simulink model "Rider_Controls_Full_CAN_Enable"  (R2014b)
settings: configuration reference "Embedded_Configuration" (kept outside this file)
PreLoadFcn:
  | load('Embedded_Config.mat')
PostLoadFcn:
  | c2000demoscallback(1)
model workspace: external: MAT-File Embedded_Config.mat (data not in the file)
libraries: canmsglib x2, c280xlib x2
settings Model: Creator=The MathWorks Inc.  LastModifiedBy=Sean

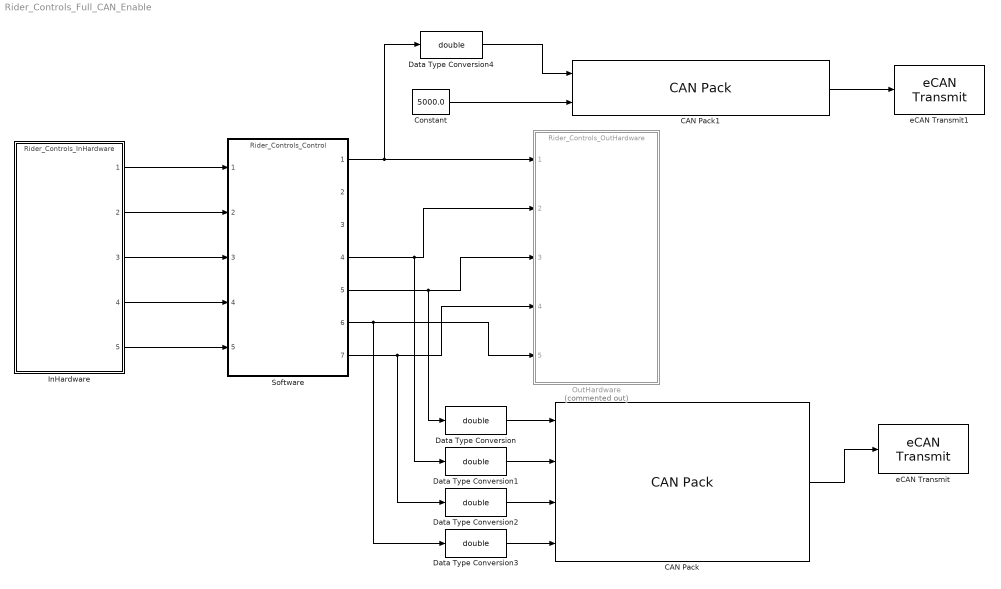
== system Rider_Controls_Full_CAN_Enable ==
  CAN Pack : canmsglib/CAN Pack  CANdbFile=C:\Users\Sean\Desktop\Buckeye Current\Databases\RW3.dbc  MsgList=DriveControlsLimits  MsgName=DriveControlsLimits  MsgIDType=Standard (11-bit identifier)  MsgIdentifier=483  MsgLength=8  SignalInfo=BatteryLimit$1$1$1$2$1$0$1$0$0$1$#RPMLimit$2$1$1$2$1$0$1$0$0$1$#StatusLimit$3$1$1$2$1$0$1$0$-Inf$Inf$#ThrottleLock$0$1$1$2$1$0$1$0$-Inf$Inf$#  NSignals=4  StartBits=str2num('[int32(1);int32(2);int32(3);int32(0)]')  SignalSizes=str2num('[int32(1);int32(1);int32(1);int32(1)]')  ByteOrders=str2num('[int32(1);int32(1);int32(1);int32(1)]')  DataTypes=str2num('[int32(2);int32(2);int32(2);int32(2)]')  MultiplexTypes=str2num('[int32(1);int32(1);int32(1);int32(1)]')  MultiplexValues=str2num('[double(0);double(0);double(0);double(0)]')  Factors=str2num('[double(1);double(1);double(1);double(1)]')  Offsets=str2num('[double(0);double(0);double(0);double(0)]')  Minimums=str2num('[double(0);double(0);double(-Inf);double(-Inf)]')  Maximums=str2num('[double(1);double(1);double(Inf);double(Inf)]')  Remote=off
      settings: DataFormat=CANdb specified signals
  CAN Pack1 : canmsglib/CAN Pack  CANdbFile=C:\Users\Sean\Desktop\Buckeye Current\Databases\RW3.dbc  MsgList=MotorDriveCommand  MsgName=MotorDriveCommand  MsgIDType=Standard (11-bit identifier)  MsgIdentifier=480  MsgLength=8  SignalInfo=MotorCurrentSetpoint$32$32$1$3$1$0$1$0$0$1$#MotorRPMSetpoint$0$32$1$3$1$0$1$0$0$4000$#  NSignals=2  StartBits=str2num('[int32(32);int32(0)]')  SignalSizes=str2num('[int32(32);int32(32)]')  ByteOrders=str2num('[int32(1);int32(1)]')  DataTypes=str2num('[int32(3);int32(3)]')  MultiplexTypes=str2num('[int32(1);int32(1)]')  MultiplexValues=str2num('[double(0);double(0)]')  Factors=str2num('[double(1);double(1)]')  Offsets=str2num('[double(0);double(0)]')  Minimums=str2num('[double(0);double(0)]')  Maximums=str2num('[double(1);double(4000)]')  Remote=off
      settings: DataFormat=CANdb specified signals
  Constant : Constant  Value=5000.0  OutDataTypeStr=Inherit: Inherit via back propagation  SampleTime=0.01
  Data Type Conversion{,1..4} (5 alike) : DataTypeConversion  OutDataTypeStr=double
  InHardware : ModelReference  ModelNameDialog=Rider_Controls_InHardware.slx  SimulationMode=Normal  ModelReferenceVersion=1.232  CopyOfModelName=Rider_Controls_InHardware.slx  DefaultDataLogging=on
  OutHardware : ModelReference  Commented=on  ModelNameDialog=Rider_Controls_OutHardware.slx  SimulationMode=Normal  ModelReferenceVersion=1.125  CopyOfModelName=Rider_Controls_OutHardware.slx  DefaultDataLogging=on
  Software : ModelReference  ModelNameDialog=Rider_Controls_Control.slx  SimulationMode=Normal  ModelReferenceVersion=1.162  CopyOfModelName=Rider_Controls_Control.slx  DefaultDataLogging=on
  eCAN Transmit : c280xlib/eCAN Transmit  chipFamily=C280x  useModule=eCAN_A  mailboxNo=31  messageID=483  messageType=Standard (11-bit identifier)  enableBlockingMode=off  postInterrupt=off  interruptLine=0
  eCAN Transmit1 : c280xlib/eCAN Transmit  chipFamily=C280x  useModule=eCAN_A  mailboxNo=30  messageID=480  messageType=Standard (11-bit identifier)  enableBlockingMode=off  postInterrupt=off  interruptLine=0
  wires:
  InHardware/1 -> Software/1
  Software/1 -> Data Type Conversion4/1, OutHardware/1
  InHardware/2 -> Software/2
  InHardware/3 -> Software/3
  InHardware/4 -> Software/4
  Software/4 -> Data Type Conversion1/1, OutHardware/2
  Software/5 -> Data Type Conversion/1, OutHardware/3
  InHardware/5 -> Software/5
  Software/7 -> Data Type Conversion2/1, OutHardware/4
  Software/6 -> Data Type Conversion3/1, OutHardware/5
  CAN Pack/1 -> eCAN Transmit/1
  Data Type Conversion/1 -> CAN Pack/1
  Data Type Conversion1/1 -> CAN Pack/2
  Data Type Conversion2/1 -> CAN Pack/3
  Data Type Conversion3/1 -> CAN Pack/4
  Constant/1 -> CAN Pack1/2
  Data Type Conversion4/1 -> CAN Pack1/1
  CAN Pack1/1 -> eCAN Transmit1/1
